simulink model "aar_generator"  (R2023a)
settings: Solver=FixedStepAuto  StartTime=0.0  StopTime=10  FixedStep=0.0001  RelTol=1e-3  AbsTol=1e-3
InitFcn:
  | addpath(fullfile(matlabroot,'toolbox/physmod/sm/sli/m'))
model workspace (MAT data in the model file):
  battery_cap = 1e-09
  contingency_time = 2
  final_demand = 1
  inertia_const = 0
  initial_amp = 0.91151
  max_torque = 1.1
  response_time = 0.05
  solar_cap = 1
  transmission_lim = 1000
undefined symbols (not defined in the file or in its folder): ee
libraries: fl_lib x141, ee_lib x60, nesl_utility x37, eeTransforms x12, batteryecm_lib x6, slpidlib x6, eeGeneralControl x6, eeSmAC1C x3, simulink x3, spsPLL3phLib x3
(part 3 of 4)

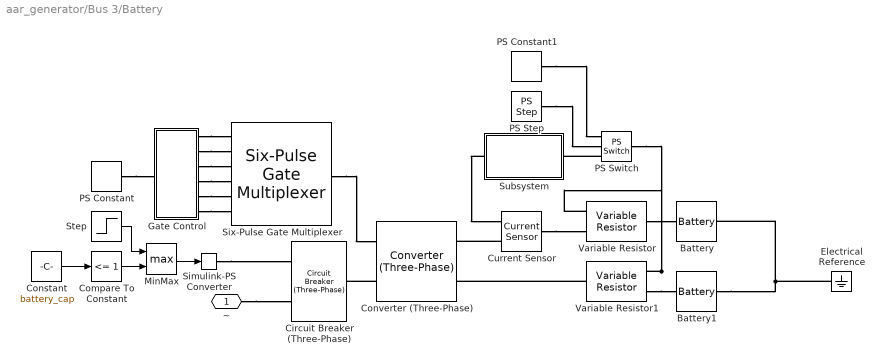
== system aar_generator/Bus 3/Battery ==
  Battery : batteryecm_lib/Battery  Vnom=494.97+50 kV  prm_dir=simscape.enum.battery.prm_dir.disabled  R1_dis=2 Ohm  R1_ch=2 Ohm  R1=0.17 Ohm  prm_AH=simscape.enum.battery.prm_AH.infinite  AH=50 A*hr  V1=11.5 V  AH1=25 A*hr  prm_R2=simscape.enum.battery.prm_R2.disabled  R2=2000 Ohm  Tmeas=298.15 K  charge_measurement_port=simscape.enum.battery.enable.no  prm_dyn=simscape.enum.battery.prm_dyn.off  Rp1=0.005 Ohm  tau1=30 s  Rp2=0.005 Ohm  tau2=30 s  Rp3=0.005 Ohm  tau3=30 s  Rp4=0.005 Ohm  tau4=30 s  Rp5=0.005 Ohm  tau5=30 s  prm_fade=simscape.enum.battery.prm_fade.disabled  N_fade=100  AH_fade=45 A*hr  R1_fade=2.02 Ohm  R1_ch_fade=2.02 Ohm  V1_fade=10.35 V  prm_age=simscape.enum.battery.prm_age.disabled  prm_age_OCV=simscape.enum.battery.prm_age_OCV.OCV  OCV_age=0.9  SOC_age=60  Tmeas_age=298.15 K  delta_time_age_vec=[0] d  temperature_age_vec=[273] K  OCV_scaling_age=2.2134e6  OCV_offset_age=1.632e6  temp_exp_age=0.515833569 V  t_exp_age=0.75  Vnom_T2=12 V  R1_T2=2.2 Ohm  R1_T2_dis=2.2 Ohm  R1_T2_ch=2.2 Ohm  V1_T2=11.4 V  R2_T2=2200 Ohm  Rp1_T2=0.005 Ohm  tau1_T2=30 s  Rp2_T2=0.005 Ohm  tau2_T2=30 s  Rp3_T2=0.005 Ohm  tau3_T2=30 s  Rp4_T2=0.005 Ohm  tau4_T2=30 s  Rp5_T2=0.005 Ohm  tau5_T2=30 s  Tmeas2=273.15 K  thermal_port=simscape.enum.thermaleffects.omit  thermal_mass=30000 J/K  i_specify=off  i_priority=None  i=0 A  i_nominal_specify=off  i_nominal_unit=A  i_nominal_value=1  v_specify=off  v_priority=None  v=0 V  v_nominal_specify=off  v_nominal_unit=V  v_nominal_value=1  charge_specify=off  charge_priority=High  charge=50 A*hr  charge_nominal_specify=off  charge_nominal_unit=A*hr  charge_nominal_value=1  num_cycles_specify=off  num_cycles_priority=High  num_cycles=0  num_cycles_nominal_specify=off  num_cycles_nominal_unit=1  num_cycles_nominal_value=1  temperature_specify=off  temperature_priority=High  temperature=298.15 K  temperature_nominal_specify=off  temperature_nominal_unit=K  temperature_nominal_value=1
  Battery1 : batteryecm_lib/Battery  Vnom=494.97+50 kV  prm_dir=simscape.enum.battery.prm_dir.disabled  R1_dis=2 Ohm  R1_ch=2 Ohm  R1=0.17 Ohm  prm_AH=simscape.enum.battery.prm_AH.infinite  AH=50 A*hr  V1=11.5 V  AH1=25 A*hr  prm_R2=simscape.enum.battery.prm_R2.disabled  R2=2000 Ohm  Tmeas=298.15 K  charge_measurement_port=simscape.enum.battery.enable.no  prm_dyn=simscape.enum.battery.prm_dyn.off  Rp1=0.005 Ohm  tau1=30 s  Rp2=0.005 Ohm  tau2=30 s  Rp3=0.005 Ohm  tau3=30 s  Rp4=0.005 Ohm  tau4=30 s  Rp5=0.005 Ohm  tau5=30 s  prm_fade=simscape.enum.battery.prm_fade.disabled  N_fade=100  AH_fade=45 A*hr  R1_fade=2.02 Ohm  R1_ch_fade=2.02 Ohm  V1_fade=10.35 V  prm_age=simscape.enum.battery.prm_age.disabled  prm_age_OCV=simscape.enum.battery.prm_age_OCV.OCV  OCV_age=0.9  SOC_age=60  Tmeas_age=298.15 K  delta_time_age_vec=[0] d  temperature_age_vec=[273] K  OCV_scaling_age=2.2134e6  OCV_offset_age=1.632e6  temp_exp_age=0.515833569 V  t_exp_age=0.75  Vnom_T2=12 V  R1_T2=2.2 Ohm  R1_T2_dis=2.2 Ohm  R1_T2_ch=2.2 Ohm  V1_T2=11.4 V  R2_T2=2200 Ohm  Rp1_T2=0.005 Ohm  tau1_T2=30 s  Rp2_T2=0.005 Ohm  tau2_T2=30 s  Rp3_T2=0.005 Ohm  tau3_T2=30 s  Rp4_T2=0.005 Ohm  tau4_T2=30 s  Rp5_T2=0.005 Ohm  tau5_T2=30 s  Tmeas2=273.15 K  thermal_port=simscape.enum.thermaleffects.omit  thermal_mass=30000 J/K  i_specify=off  i_priority=None  i=0 A  i_nominal_specify=off  i_nominal_unit=A  i_nominal_value=1  v_specify=off  v_priority=None  v=0 V  v_nominal_specify=off  v_nominal_unit=V  v_nominal_value=1  charge_specify=off  charge_priority=High  charge=50 A*hr  charge_nominal_specify=off  charge_nominal_unit=A*hr  charge_nominal_value=1  num_cycles_specify=off  num_cycles_priority=High  num_cycles=0  num_cycles_nominal_specify=off  num_cycles_nominal_unit=1  num_cycles_nominal_value=1  temperature_specify=off  temperature_priority=High  temperature=298.15 K  temperature_nominal_specify=off  temperature_nominal_unit=K  temperature_nominal_value=1
  Circuit Breaker (Three-Phase) : ee_lib/Switches & Breakers/Circuit Breaker (Three-Phase)  R_closed=1e-9 Ohm  G_open=1e-9 1/Ohm  threshold=0.5 V  breaker_behavior=ee.enum.switches.breakerBehavior.zeroCrossingEnable
      settings: InternalSimscapePortConfiguration="{\"Bottom\":[],\"Left\":[{\"id\":\"vT\",\"label\":\"vT\",\"type\":\"input\"},{\"id\":\"N1\",\"label\":\"~1\",\"type\":\"foundation.electrical.three_phase\"}],\"Right\":[{\"id\":\"N2\",\"label\":\"~2\",\"type\":\"foundation.electrical.three_phase\"}],\"Top\":[]}"
  Compare To Constant : simulink/Logic and Bit Operations/Compare To Constant  relop=<=  const=1  OutDataTypeStr=uint8
  Constant : Constant  Value=battery_cap
  Converter (Three-Phase) : ee_lib/Semiconductors & Converters/Converters/Converter (Three-Phase)  port_option=ee.enum.threePhasePort.composite  device_type=ee.enum.converters.switchingdevice.averaged  K=0  Vf=0.8 V  Ron=1e-9 mOhm  Rds=0.001 Ohm  Goff=1e-6 1/Ohm  Vgt=1 V  Vgt_off=-1 V  Ih=1 A  Vth=6 V  diode_param=ee.enum.converters.protectiondiode.none  diode_Vf=1 MV  diode_Ron=0.001 Ohm  diode_Goff=1e-5 1/Ohm  diode_C=50 nF  diode_iRM=-235 A  diode_iF=300 A  diode_idot=-50 A/us  diode_trr_param=ee.enum.converters.diodetrr.trr_factor  diode_trr_factor=3  diode_trr=15 us  diode_Qrr=1500 s*uA  snubber_type=ee.enum.converters.snubber.exclude  Cs=1e-7 F  Rs=0.1 Ohm
  Current Sensor : fl_lib/Electrical/Electrical Sensors/Current Sensor
  Electrical Reference : fl_lib/Electrical/Electrical Elements/Electrical Reference
  Gate Control : Subsystem
  MinMax : MinMax  Function=max  Inputs=2
  PS Constant : fl_lib/Physical Signals/Sources/PS Constant  constant=1
  PS Constant1 : fl_lib/Physical Signals/Sources/PS Constant  constant=0 Ohm
  PS Step : fl_lib/Physical Signals/Sources/PS Step  step_time=0.00025 s  initial_value=1  final_value=0
  PS Switch : fl_lib/Physical Signals/Nonlinear Operators/PS Switch  Threshold=0.5
      settings: InternalSimscapePortConfiguration="{\"Bottom\":[],\"Left\":[{\"id\":\"I1\",\"label\":\"\",\"type\":\"input\"},{\"id\":\"I2\",\"label\":\"\",\"type\":\"input\"},{\"id\":\"I3\",\"label\":\"\",\"type\":\"input\"}],\"Right\":[{\"id\":\"O\",\"label\":\"\",\"type\":\"output\"}],\"Top\":[]}"
  Simulink-PS Converter : nesl_utility/Simulink-PS Converter  PhysicalDomain=network_engine_domain  SubClassName=ps_input  LeftPortType=input  RightPortType=output  PseudoPeriodic=off  Frequencies=[]  NoiseDistribution=none  NoiseParameters=[]  Unit=V  AffineConversion=off  FilteringAndDerivatives=provide  SimscapeFilterOrder=1  InputFilterTimeConstant=0.001  UdotUserProvided=0
  Six-Pulse Gate Multiplexer : ee_lib/Semiconductors & Converters/Converters/Six-Pulse Gate Multiplexer  port_option=ee.enum.controlport.ps
  Step : Step  Time=contingency_time+response_time  Before=1  After=0  SampleTime=0
  Subsystem : Subsystem
  Variable Resistor : fl_lib/Electrical/Electrical Elements/Variable Resistor  Rmin=0 Ohm  i_specify=off  i_priority=None  i=0 A  i_nominal_specify=off  i_nominal_unit=A  i_nominal_value=1  v_specify=off  v_priority=None  v=0 V  v_nominal_specify=off  v_nominal_unit=V  v_nominal_value=1
  Variable Resistor1 : fl_lib/Electrical/Electrical Elements/Variable Resistor  Rmin=0 Ohm  i_specify=off  i_priority=None  i=0 A  i_nominal_specify=off  i_nominal_unit=A  i_nominal_value=1  v_specify=off  v_priority=None  v=0 V  v_nominal_specify=off  v_nominal_unit=V  v_nominal_value=1
  ~ : PMIOPort  Side=Left
  wires:
  Constant/1 -> Compare To Constant/1
  MinMax/1 -> Simulink-PS Converter/1
  Step/1 -> MinMax/1
  Compare To Constant/1 -> MinMax/2
  connections:
  PS Constant1/RConn1 -- PS Switch/LConn1
  PS Step/RConn1 -- PS Switch/LConn2
  Variable Resistor1/LConn1 -- Variable Resistor/LConn1 -- PS Switch/RConn1
  PS Switch/LConn3 -- Subsystem/RConn1
  Simulink-PS Converter/RConn1 -- Circuit Breaker (Three-Phase)/LConn1
  ~/RConn1 -- Circuit Breaker (Three-Phase)/LConn2
  Converter (Three-Phase)/LConn2 -- Circuit Breaker (Three-Phase)/RConn1
  Subsystem/LConn1 -- Current Sensor/RConn1
  Current Sensor/LConn1 -- Variable Resistor/LConn2
  Variable Resistor1/LConn2 -- Battery1/RConn1
  Variable Resistor1/RConn1 -- Converter (Three-Phase)/RConn2
  Variable Resistor/RConn1 -- Battery/LConn1
  Current Sensor/RConn2 -- Converter (Three-Phase)/RConn1
  Electrical Reference/LConn1 -- Battery/RConn1 -- Battery1/LConn1
  PS Constant/RConn1 -- Gate Control/LConn1
  Gate Control/RConn6 -- Six-Pulse Gate Multiplexer/LConn6
  Gate Control/RConn5 -- Six-Pulse Gate Multiplexer/LConn5
  Gate Control/RConn4 -- Six-Pulse Gate Multiplexer/LConn4
  Gate Control/RConn3 -- Six-Pulse Gate Multiplexer/LConn3
  Gate Control/RConn2 -- Six-Pulse Gate Multiplexer/LConn2
  Gate Control/RConn1 -- Six-Pulse Gate Multiplexer/LConn1
  Six-Pulse Gate Multiplexer/RConn1 -- Converter (Three-Phase)/LConn1

== system aar_generator/Bus 3/Governor and Prime Mover ==
  Governor : Subsystem
  Ideal Torque Source : fl_lib/Mechanical/Mechanical Sources/Ideal Torque Source
  Mechanical Rotational Reference : fl_lib/Mechanical/Rotational Elements/Mechanical Rotational Reference
  Non-reheat turbine : Subsystem
  PS-Simulink Converter : nesl_utility/PS-Simulink Converter  PhysicalDomain=network_engine_domain  SubClassName=ps_output  LeftPortType=input  RightPortType=output  PseudoPeriodic=off  Frequencies=[]  VectorFormat=1-D array  Unit=1  AffineConversion=off
  Rotor Velocity Measurement : ee_lib/Electromechanical/Synchronous/Synchronous Machine Measurement  output_idx=4
      settings: InternalSimscapePortConfiguration="{\"Bottom\":[],\"Left\":[{\"id\":\"pu_input\",\"label\":\"pu\",\"type\":\"input\"}],\"Right\":[{\"id\":\"pu_output\",\"label\":\"o\",\"type\":\"output\"}],\"Top\":[]}"
  Simulink-PS Converter : nesl_utility/Simulink-PS Converter  PhysicalDomain=network_engine_domain  SubClassName=ps_input  LeftPortType=input  RightPortType=output  PseudoPeriodic=off  Frequencies=[]  NoiseDistribution=none  NoiseParameters=[]  Unit=1  AffineConversion=off  FilteringAndDerivatives=zero  SimscapeFilterOrder=1  InputFilterTimeConstant=0.001  UdotUserProvided=1
  scale by base_torque : Gain  Gain=base_torque
  R : PMIOPort  Side=Right
  C : PMIOPort  Port=2  Side=Right
  pu : PMIOPort  Port=3  Side=Left
  wires:
  Non-reheat turbine/1(torque) -> scale by base_torque/1
  scale by base_torque/1 -> Simulink-PS Converter/1
  Governor/1(delta_y) -> Non-reheat turbine/1(delta_y)
  PS-Simulink Converter/1 -> Governor/1(pu_velocity)
  connections:
  Simulink-PS Converter/RConn1 -- Ideal Torque Source/RConn1
  PS-Simulink Converter/LConn1 -- Rotor Velocity Measurement/RConn1
  pu/RConn1 -- Rotor Velocity Measurement/LConn1
  Ideal Torque Source/LConn1 -- R/RConn1
  Mechanical Rotational Reference/LConn1 -- Ideal Torque Source/RConn2 -- C/RConn1

== system aar_generator/Bus 3/Load Control ==
  PS Gain : fl_lib/Physical Signals/Functions/PS Gain  gain=load MW
  PS Min : fl_lib/Physical Signals/Nonlinear Operators/PS Min
      settings: InternalSimscapePortConfiguration="{\"Bottom\":[],\"Left\":[{\"id\":\"I1\",\"label\":\"\",\"type\":\"input\"},{\"id\":\"I2\",\"label\":\"\",\"type\":\"input\"}],\"Right\":[{\"id\":\"O\",\"label\":\"\",\"type\":\"output\"}],\"Top\":[]}"
  PS Step : fl_lib/Physical Signals/Sources/PS Step  step_time=contingency_time+response_time s  initial_value=1  final_value=final_demand
  PS Step1 : fl_lib/Physical Signals/Sources/PS Step  step_time=0.15 s  initial_value=0.2  final_value=1
  Load (MW) : PMIOPort  Side=Right
  connections:
  PS Step1/RConn1 -- PS Min/LConn1
  PS Step/RConn1 -- PS Min/LConn2
  PS Min/RConn1 -- PS Gain/LConn1
  PS Gain/RConn1 -- Load (MW)/RConn1

== system aar_generator/Bus 3/Solar Panel ==
  Controlled Current Source (Three-Phase) : ee_lib/Sources/Controlled Current Source (Three-Phase)  input_option=ee.enum.inputType.instantaneous  FRated=60 Hz
      settings: InternalSimscapePortConfiguration="{\"Bottom\":[],\"Left\":[{\"id\":\"S\",\"label\":\"S\",\"type\":\"input\"},{\"id\":\"n\",\"label\":\"n\",\"type\":\"foundation.electrical.electrical\"}],\"Right\":[{\"id\":\"N\",\"label\":\"~\",\"type\":\"foundation.electrical.three_phase\"}],\"Top\":[]}"
  Current Control : Subsystem
  Electrical Reference : fl_lib/Electrical/Electrical Elements/Electrical Reference
  Grounded Neutral (Three-Phase) : ee_lib/Connectors & References/Grounded Neutral (Three-Phase)
  PS Step : fl_lib/Physical Signals/Sources/PS Step  step_time=0.15 s  initial_value=0  final_value=1
  Power Control : Subsystem
  Power Sensor (Three-Phase) : ee_lib/Sensors & Transducers/Power Sensor (Three-Phase)  load_type=ee.enum.passive.type_balanced.balanced  f0=60 Hz  config=ee.enum.with_neutral.no  rho=1
      settings: InternalSimscapePortConfiguration="{\"Bottom\":[],\"Left\":[{\"id\":\"N1\",\"label\":\"~1\",\"type\":\"foundation.electrical.three_phase\"}],\"Right\":[{\"id\":\"N2\",\"label\":\"~2\",\"type\":\"foundation.electrical.three_phase\"}],\"Top\":[{\"id\":\"Pm\",\"label\":\"P\",\"type\":\"output\"},{\"id\":\"Qm\",\"label\":\"Q\",\"type\":\"output\"}]}"
  SI to pu : Gain  Gain=1/(350*sqrt(2)*10^3)
  SPDT Switch (Three-Phase) : ee_lib/Switches & Breakers/SPDT Switch (Three-Phase)  R_closed=0.001 Ohm  G_open=1e-6 1/Ohm  threshold=0.5 V  i_vT_specify=off  i_vT_priority=None  i_vT=0 A  i_vT_nominal_specify=off  i_vT_nominal_unit=A  i_vT_nominal_value=1  I12_specify=off  I12_priority=None  I12=[0, 0, 0] A  I12_nominal_specify=off  I12_nominal_unit=A  I12_nominal_value=1  V12_specify=off  V12_priority=None  V12=[0, 0, 0] V  V12_nominal_specify=off  V12_nominal_unit=V  V12_nominal_value=1  I13_specify=off  I13_priority=None  I13=[0, 0, 0] A  I13_nominal_specify=off  I13_nominal_unit=A  I13_nominal_value=1  V13_specify=off  V13_priority=None  V13=[0, 0, 0] V  V13_nominal_specify=off  V13_nominal_unit=V  V13_nominal_value=1  i_a_12_specify=off  i_a_12_priority=None  i_a_12=0 A  i_a_12_nominal_specify=off  i_a_12_nominal_unit=A  i_a_12_nominal_value=1  v_a_12_specify=off  v_a_12_priority=None  v_a_12=0 V  v_a_12_nominal_specify=off  v_a_12_nominal_unit=V  v_a_12_nominal_value=1  i_a_13_specify=off  i_a_13_priority=None  i_a_13=0 A  i_a_13_nominal_specify=off  i_a_13_nominal_unit=A  i_a_13_nominal_value=1  v_a_13_specify=off  v_a_13_priority=None  v_a_13=0 V  v_a_13_nominal_specify=off  v_a_13_nominal_unit=V  v_a_13_nominal_value=1  i_b_12_specify=off  i_b_12_priority=None  i_b_12=0 A  i_b_12_nominal_specify=off  i_b_12_nominal_unit=A  i_b_12_nominal_value=1  v_b_12_specify=off  v_b_12_priority=None  v_b_12=0 V  v_b_12_nominal_specify=off  v_b_12_nominal_unit=V  v_b_12_nominal_value=1  i_b_13_specify=off  i_b_13_priority=None  i_b_13=0 A  i_b_13_nominal_specify=off  i_b_13_nominal_unit=A  i_b_13_nominal_value=1  v_b_13_specify=off  v_b_13_priority=None  v_b_13=0 V  v_b_13_nominal_specify=off  v_b_13_nominal_unit=V  v_b_13_nominal_value=1  i_c_12_specify=off  i_c_12_priority=None  i_c_12=0 A  i_c_12_nominal_specify=off  i_c_12_nominal_unit=A  i_c_12_nominal_value=1  v_c_12_specify=off  v_c_12_priority=None  v_c_12=0 V  v_c_12_nominal_specify=off  v_c_12_nominal_unit=V  v_c_12_nominal_value=1  i_c_13_specify=off  i_c_13_priority=None  i_c_13=0 A  i_c_13_nominal_specify=off  i_c_13_nominal_unit=A  i_c_13_nominal_value=1  v_c_13_specify=off  v_c_13_priority=None  v_c_13=0 V  v_c_13_nominal_specify=off  v_c_13_nominal_unit=V  v_c_13_nominal_value=1
      settings: InternalSimscapePortConfiguration="{\"Bottom\":[],\"Left\":[{\"id\":\"vT\",\"label\":\"vT\",\"type\":\"input\"},{\"id\":\"N1\",\"label\":\"~1\",\"type\":\"foundation.electrical.three_phase\"}],\"Right\":[{\"id\":\"N2\",\"label\":\"~2\",\"type\":\"foundation.electrical.three_phase\"},{\"id\":\"N3\",\"label\":\"~3\",\"type\":\"foundation.electrical.three_phase\"}],\"Top\":[]}"
  ~ : PMIOPort  Side=Left
  wires:
  [Phase3] -> Current Control/3(Phase)
  Power Control/2(Qset (pu)) -> Current Control/2(Qset (pu))
  [Freq3] -> Power Control/1(Freq (Hz))
  Power Control/1(Pset (pu)) -> Current Control/1(Pset (pu))
  [V3] -> SI to pu/1
  SI to pu/1 -> Current Control/4(Vabc (pu))
  connections:
  Current Control/RConn1 -- Controlled Current Source (Three-Phase)/LConn1
  Electrical Reference/LConn1 -- Controlled Current Source (Three-Phase)/LConn2
  Power Sensor (Three-Phase)/LConn1 -- Controlled Current Source (Three-Phase)/RConn1
  Power Control/LConn1 -- Power Sensor (Three-Phase)/LConn3
  ~/RConn1 -- SPDT Switch (Three-Phase)/RConn2
  PS Step/RConn1 -- SPDT Switch (Three-Phase)/LConn1
  SPDT Switch (Three-Phase)/LConn2 -- Power Sensor (Three-Phase)/RConn1
  Grounded Neutral (Three-Phase)/LConn1 -- SPDT Switch (Three-Phase)/RConn1

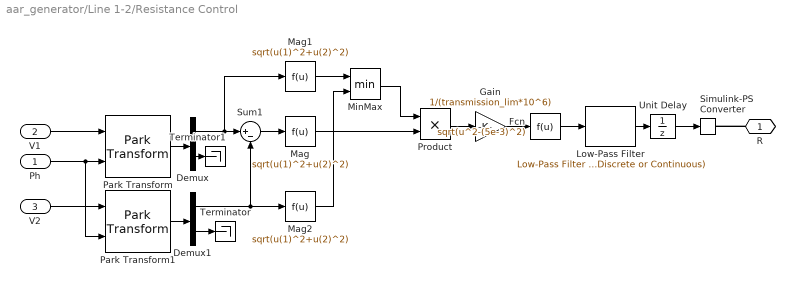
== system aar_generator/Line 1-2/Resistance Control ==
  Ph : Inport
  V1 : Inport  Port=2
  V2 : Inport  Port=3
  Demux : Demux  Outputs=[2 1]
  Demux1 : Demux  Outputs=[2 1]
  Fcn : Fcn  Expr=sqrt(u^2-(5e-3)^2)
  Gain : Gain  Gain=1/(transmission_lim*10^6)
  Low-Pass Filter : eeGeneralControl/Low-Pass Filter (Discrete or Continuous)  K=1  T=0.1  B=inf  A=-inf  init_option=Inherited from block input  x0=0  Ts=-1
  Mag : Fcn  Expr=sqrt(u(1)^2+u(2)^2)
  Mag1 : Fcn  Expr=sqrt(u(1)^2+u(2)^2)
  Mag2 : Fcn  Expr=sqrt(u(1)^2+u(2)^2)
  MinMax : MinMax  Inputs=2
  Park Transform : eeTransforms/Park Transform  AxisAlignment=Q-axis  PowerInvariant=off
      settings: LibrarySourceBlock=|
      | ee_sl_lib/Mathematical
      | Transforms/Park Transform
  Park Transform1 : eeTransforms/Park Transform  AxisAlignment=Q-axis  PowerInvariant=off
      settings: LibrarySourceBlock=|
      | ee_sl_lib/Mathematical
      | Transforms/Park Transform
  Product : Product
  Simulink-PS Converter : nesl_utility/Simulink-PS Converter  PhysicalDomain=network_engine_domain  SubClassName=ps_input  LeftPortType=input  RightPortType=output  PseudoPeriodic=off  Frequencies=[]  NoiseDistribution=none  NoiseParameters=[]  Unit=Ohm  AffineConversion=off  FilteringAndDerivatives=provide  SimscapeFilterOrder=1  InputFilterTimeConstant=0.001  UdotUserProvided=0
  Sum1 : Sum  Inputs=|+-
  Terminator : Terminator
  Terminator1 : Terminator
  Unit Delay : UnitDelay  SampleTime=-1  HasFrameUpgradeWarning=on
  R : PMIOPort  Side=Right
  wires:
  Unit Delay/1 -> Simulink-PS Converter/1
  V1/1 -> Park Transform/1
  V2/1 -> Park Transform1/1
  Ph/1 -> Park Transform1/2, Park Transform/2
  Park Transform/1 -> Demux/1
  Park Transform1/1 -> Demux1/1
  Demux1/2 -> Terminator/1
  Demux/2 -> Terminator1/1
  Demux/1 -> Mag1/1, Sum1/1
  Demux1/1 -> Mag2/1, Sum1/2
  Sum1/1 -> Mag/1
  Mag1/1 -> MinMax/1
  Mag2/1 -> MinMax/2
  Mag/1 -> Product/2
  MinMax/1 -> Product/1
  Product/1 -> Gain/1
  Low-Pass Filter/1 -> Unit Delay/1
  Gain/1 -> Fcn/1
  Fcn/1 -> Low-Pass Filter/1
  connections:
  R/RConn1 -- Simulink-PS Converter/RConn1

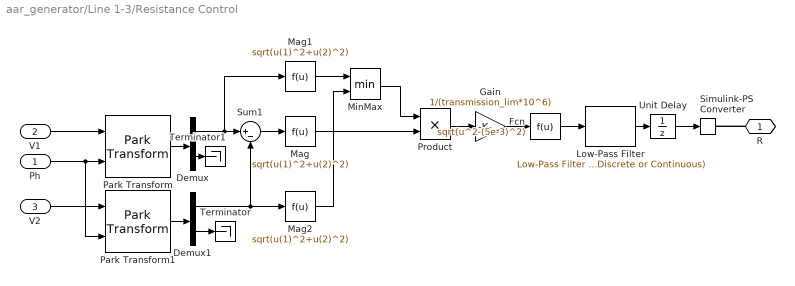
== system aar_generator/Line 1-3/Resistance Control ==
  Ph : Inport
  V1 : Inport  Port=2
  V2 : Inport  Port=3
  Demux : Demux  Outputs=[2 1]
  Demux1 : Demux  Outputs=[2 1]
  Fcn : Fcn  Expr=sqrt(u^2-(5e-3)^2)
  Gain : Gain  Gain=1/(transmission_lim*10^6)
  Low-Pass Filter : eeGeneralControl/Low-Pass Filter (Discrete or Continuous)  K=1  T=0.1  B=inf  A=-inf  init_option=Inherited from block input  x0=0  Ts=-1
  Mag : Fcn  Expr=sqrt(u(1)^2+u(2)^2)
  Mag1 : Fcn  Expr=sqrt(u(1)^2+u(2)^2)
  Mag2 : Fcn  Expr=sqrt(u(1)^2+u(2)^2)
  MinMax : MinMax  Inputs=2
  Park Transform : eeTransforms/Park Transform  AxisAlignment=Q-axis  PowerInvariant=off
      settings: LibrarySourceBlock=|
      | ee_sl_lib/Mathematical
      | Transforms/Park Transform
  Park Transform1 : eeTransforms/Park Transform  AxisAlignment=Q-axis  PowerInvariant=off
      settings: LibrarySourceBlock=|
      | ee_sl_lib/Mathematical
      | Transforms/Park Transform
  Product : Product
  Simulink-PS Converter : nesl_utility/Simulink-PS Converter  PhysicalDomain=network_engine_domain  SubClassName=ps_input  LeftPortType=input  RightPortType=output  PseudoPeriodic=off  Frequencies=[]  NoiseDistribution=none  NoiseParameters=[]  Unit=Ohm  AffineConversion=off  FilteringAndDerivatives=provide  SimscapeFilterOrder=1  InputFilterTimeConstant=0.001  UdotUserProvided=0
  Sum1 : Sum  Inputs=|+-
  Terminator : Terminator
  Terminator1 : Terminator
  Unit Delay : UnitDelay  SampleTime=-1  HasFrameUpgradeWarning=on
  R : PMIOPort  Side=Right
  wires:
  Unit Delay/1 -> Simulink-PS Converter/1
  V1/1 -> Park Transform/1
  V2/1 -> Park Transform1/1
  Ph/1 -> Park Transform1/2, Park Transform/2
  Park Transform/1 -> Demux/1
  Park Transform1/1 -> Demux1/1
  Demux1/2 -> Terminator/1
  Demux/2 -> Terminator1/1
  Demux/1 -> Mag1/1, Sum1/1
  Demux1/1 -> Mag2/1, Sum1/2
  Sum1/1 -> Mag/1
  Mag1/1 -> MinMax/1
  Mag2/1 -> MinMax/2
  Mag/1 -> Product/2
  MinMax/1 -> Product/1
  Product/1 -> Gain/1
  Low-Pass Filter/1 -> Unit Delay/1
  Gain/1 -> Fcn/1
  Fcn/1 -> Low-Pass Filter/1
  connections:
  R/RConn1 -- Simulink-PS Converter/RConn1

== system aar_generator/Line 2-3/Resistance Control ==
  Ph : Inport
  V1 : Inport  Port=2
  V2 : Inport  Port=3
  Demux : Demux  Outputs=[2 1]
  Demux1 : Demux  Outputs=[2 1]
  Fcn : Fcn  Expr=sqrt(u^2-(5e-3)^2)
  Gain : Gain  Gain=1/(transmission_lim*10^6)
  Low-Pass Filter : eeGeneralControl/Low-Pass Filter (Discrete or Continuous)  K=1  T=0.1  B=inf  A=-inf  init_option=Inherited from block input  x0=0  Ts=-1
  Mag : Fcn  Expr=sqrt(u(1)^2+u(2)^2)
  Mag1 : Fcn  Expr=sqrt(u(1)^2+u(2)^2)
  Mag2 : Fcn  Expr=sqrt(u(1)^2+u(2)^2)
  MinMax : MinMax  Inputs=2
  Park Transform : eeTransforms/Park Transform  AxisAlignment=Q-axis  PowerInvariant=off
      settings: LibrarySourceBlock=|
      | ee_sl_lib/Mathematical
      | Transforms/Park Transform
  Park Transform1 : eeTransforms/Park Transform  AxisAlignment=Q-axis  PowerInvariant=off
      settings: LibrarySourceBlock=|
      | ee_sl_lib/Mathematical
      | Transforms/Park Transform
  Product : Product
  Simulink-PS Converter : nesl_utility/Simulink-PS Converter  PhysicalDomain=network_engine_domain  SubClassName=ps_input  LeftPortType=input  RightPortType=output  PseudoPeriodic=off  Frequencies=[]  NoiseDistribution=none  NoiseParameters=[]  Unit=Ohm  AffineConversion=off  FilteringAndDerivatives=provide  SimscapeFilterOrder=1  InputFilterTimeConstant=0.001  UdotUserProvided=0
  Sum1 : Sum  Inputs=|+-
  Terminator : Terminator
  Terminator1 : Terminator
  Unit Delay : UnitDelay  SampleTime=-1  HasFrameUpgradeWarning=on
  R : PMIOPort  Side=Right
  wires:
  Unit Delay/1 -> Simulink-PS Converter/1
  V1/1 -> Park Transform/1
  V2/1 -> Park Transform1/1
  Ph/1 -> Park Transform1/2, Park Transform/2
  Park Transform/1 -> Demux/1
  Park Transform1/1 -> Demux1/1
  Demux1/2 -> Terminator/1
  Demux/2 -> Terminator1/1
  Demux/1 -> Mag1/1, Sum1/1
  Demux1/1 -> Mag2/1, Sum1/2
  Sum1/1 -> Mag/1
  Mag1/1 -> MinMax/1
  Mag2/1 -> MinMax/2
  Mag/1 -> Product/2
  MinMax/1 -> Product/1
  Product/1 -> Gain/1
  Low-Pass Filter/1 -> Unit Delay/1
  Gain/1 -> Fcn/1
  Fcn/1 -> Low-Pass Filter/1
  connections:
  R/RConn1 -- Simulink-PS Converter/RConn1

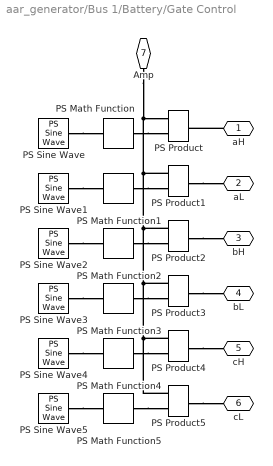
== system aar_generator/Bus 1/Battery/Gate Control ==
  PS Math Function{,1..5} (6 alike) : fl_lib/Physical Signals/Functions/PS Math Function  fcn_choice=foundation.enum.math_function.square  v=1
  PS Product{,1..5} (6 alike) : fl_lib/Physical Signals/Functions/PS Product
  PS Sine Wave : fl_lib/Physical Signals/Sources/PS Sine Wave  amplitude=1  bias=0  frequency_spec=foundation.enum.frequencySpec.frequencySI  frequency_SI=30 Hz  frequency_angular=1 rad/s  phase=pi/2 rad
      settings: InternalSimscapePortConfiguration="{\"Bottom\":[],\"Left\":[],\"Right\":[{\"id\":\"O\",\"label\":\"\",\"type\":\"output\"}],\"Top\":[]}"
  PS Sine Wave1 : fl_lib/Physical Signals/Sources/PS Sine Wave  amplitude=1  bias=0  frequency_spec=foundation.enum.frequencySpec.frequencySI  frequency_SI=30 Hz  frequency_angular=1 rad/s  phase=0 rad
      settings: InternalSimscapePortConfiguration="{\"Bottom\":[],\"Left\":[],\"Right\":[{\"id\":\"O\",\"label\":\"\",\"type\":\"output\"}],\"Top\":[]}"
  PS Sine Wave2 : fl_lib/Physical Signals/Sources/PS Sine Wave  amplitude=1  bias=0  frequency_spec=foundation.enum.frequencySpec.frequencySI  frequency_SI=30 Hz  frequency_angular=1 rad/s  phase=2*pi/3+pi/2 rad
      settings: InternalSimscapePortConfiguration="{\"Bottom\":[],\"Left\":[],\"Right\":[{\"id\":\"O\",\"label\":\"\",\"type\":\"output\"}],\"Top\":[]}"
  PS Sine Wave3 : fl_lib/Physical Signals/Sources/PS Sine Wave  amplitude=1  bias=0  frequency_spec=foundation.enum.frequencySpec.frequencySI  frequency_SI=30 Hz  frequency_angular=1 rad/s  phase=2*pi/3 rad
      settings: InternalSimscapePortConfiguration="{\"Bottom\":[],\"Left\":[],\"Right\":[{\"id\":\"O\",\"label\":\"\",\"type\":\"output\"}],\"Top\":[]}"
  PS Sine Wave4 : fl_lib/Physical Signals/Sources/PS Sine Wave  amplitude=1  bias=0  frequency_spec=foundation.enum.frequencySpec.frequencySI  frequency_SI=30 Hz  frequency_angular=1 rad/s  phase=-2*pi/3+pi/2 rad
      settings: InternalSimscapePortConfiguration="{\"Bottom\":[],\"Left\":[],\"Right\":[{\"id\":\"O\",\"label\":\"\",\"type\":\"output\"}],\"Top\":[]}"
  PS Sine Wave5 : fl_lib/Physical Signals/Sources/PS Sine Wave  amplitude=1  bias=0  frequency_spec=foundation.enum.frequencySpec.frequencySI  frequency_SI=30 Hz  frequency_angular=1 rad/s  phase=-2*pi/3 rad
      settings: InternalSimscapePortConfiguration="{\"Bottom\":[],\"Left\":[],\"Right\":[{\"id\":\"O\",\"label\":\"\",\"type\":\"output\"}],\"Top\":[]}"
  aH : PMIOPort  Side=Right
  aL : PMIOPort  Port=2  Side=Right
  bH : PMIOPort  Port=3  Side=Right
  bL : PMIOPort  Port=4  Side=Right
  cH : PMIOPort  Port=5  Side=Right
  cL : PMIOPort  Port=6  Side=Right
  Amp : PMIOPort  Port=7  Side=Left
  connections:
  aH/RConn1 -- PS Product/RConn1
  PS Math Function/RConn1 -- PS Product/LConn2
  Amp/RConn1 -- PS Product/LConn1 -- PS Product1/LConn1 -- PS Product2/LConn1 -- PS Product3/LConn1 -- PS Product5/LConn1 -- PS Product4/LConn1
  PS Sine Wave/RConn1 -- PS Math Function/LConn1
  PS Math Function1/RConn1 -- PS Product1/LConn2
  PS Sine Wave1/RConn1 -- PS Math Function1/LConn1
  PS Product1/RConn1 -- aL/RConn1
  PS Math Function2/RConn1 -- PS Product2/LConn2
  PS Sine Wave2/RConn1 -- PS Math Function2/LConn1
  PS Product2/RConn1 -- bH/RConn1
  PS Math Function3/RConn1 -- PS Product3/LConn2
  PS Sine Wave3/RConn1 -- PS Math Function3/LConn1
  PS Product3/RConn1 -- bL/RConn1
  PS Math Function4/RConn1 -- PS Product4/LConn2
  PS Sine Wave4/RConn1 -- PS Math Function4/LConn1
  PS Math Function5/RConn1 -- PS Product5/LConn2
  PS Sine Wave5/RConn1 -- PS Math Function5/LConn1
  PS Product4/RConn1 -- cH/RConn1
  PS Product5/RConn1 -- cL/RConn1

== system aar_generator/Bus 1/Battery/Subsystem ==
  Internal Resistance : fl_lib/Physical Signals/Sources/PS Constant  constant=0.34 Ohm
  PS Add : fl_lib/Physical Signals/Functions/PS Add
  PS Gain1 : fl_lib/Physical Signals/Functions/PS Gain  gain=0.5
  PS Gain2 : fl_lib/Physical Signals/Functions/PS Gain  gain=battery_cap MW
  PS Gain3 : fl_lib/Physical Signals/Functions/PS Gain  gain=2*350*sqrt(2) kV
  PS Math Function : fl_lib/Physical Signals/Functions/PS Math Function  fcn_choice=foundation.enum.math_function.square  v=1
  PS Math Function1 : fl_lib/Physical Signals/Functions/PS Math Function  fcn_choice=foundation.enum.math_function.reciprocal  v=1
  PS Subtract : fl_lib/Physical Signals/Functions/PS Subtract
  I : PMIOPort  Side=Left
  r : PMIOPort  Port=2  Side=Right
  connections:
  I/RConn1 -- PS Math Function1/LConn1
  PS Gain1/LConn1 -- PS Subtract/RConn1
  PS Gain1/RConn1 -- r/RConn1
  PS Add/RConn1 -- PS Subtract/LConn2
  Internal Resistance/RConn1 -- PS Add/LConn2
  PS Math Function1/RConn1 -- PS Math Function/LConn1 -- PS Gain3/LConn1
  PS Gain2/LConn1 -- PS Math Function/RConn1
  PS Add/LConn1 -- PS Gain2/RConn1
  PS Gain3/RConn1 -- PS Subtract/LConn1

== system aar_generator/Bus 1/Governor and Prime Mover/Governor ==
  pu_velocity : Inport
  1/T_G : Gain  Gain=1/T_G
  1/droop : Gain  Gain=1/(droop_percentage/100)
  Delta load setpoint : Sum  Inputs=+-|
  Delta speed : Sum  Inputs=-+|
  Integrator : Integrator  InitialCondition=pu_torque0
  Load_setpoint : Constant  Value=pu_load_reference_setpoint
  Speed_ref : Constant  Value=pu_speed_reference
  Subtract : Sum  Inputs=|+-
  delta_y : Outport  VectorParamsAs1DForOutWhenUnconnected=off
  wires:
  Speed_ref/1 -> Delta speed/1
  Delta speed/1 -> 1/droop/1
  Load_setpoint/1 -> Delta load setpoint/1
  pu_velocity/1 -> Delta speed/2
  1/droop/1 -> Delta load setpoint/2
  Delta load setpoint/1 -> Subtract/1
  Subtract/1 -> 1/T_G/1
  1/T_G/1 -> Integrator/1
  Integrator/1 -> delta_y/1, Subtract/2

== system aar_generator/Bus 1/Governor and Prime Mover/Non-reheat turbine ==
  delta_y : Inport
  1/T_CH : Gain  Gain=1/T_CH
  Integrator : Integrator  InitialCondition=pu_torque0  UpperSaturationLimit=max_torque
  Max : MinMax  Function=max  Inputs=2
  Min : MinMax  Inputs=2
  Step : Step  Time=contingency_time  Before=max_torque  After=contingency_torque  SampleTime=0
  Sum : Sum  Inputs=|+-
  has_contingency : Constant  Value=max_torque*(1-has_contingency)
  torque : Outport  VectorParamsAs1DForOutWhenUnconnected=off
  wires:
  delta_y/1 -> Sum/1
  Sum/1 -> 1/T_CH/1
  1/T_CH/1 -> Integrator/1
  Min/1 -> Sum/2, torque/1
  Integrator/1 -> Min/2
  Max/1 -> Min/1
  Step/1 -> Max/2
  has_contingency/1 -> Max/1

== system aar_generator/Bus 1/Solar Panel/Current Control ==
  Pset (pu) : Inport
  Qset (pu) : Inport  Port=2
  Phase : Inport  Port=3
  Vabc (pu) : Inport  Port=4
  Constant : Constant  Value=0
  Demux : Demux  Outputs=[2 1]
  Divide : Product  Inputs=*/
  Id : Fcn  Expr=u(1)*u(3)+u(2)*u(4)
  Inverse Park Transform : eeTransforms/Inverse Park Transform  AxisAlignment=Q-axis  PowerInvariant=off
      settings: LibrarySourceBlock=|
      | ee_sl_lib/Mathematical
      | Transforms/Inverse
      | Park Transform
  Iq : Fcn  Expr=u(1)*u(4)-u(2)*u(3)
  Mag^2 : Fcn  Expr=u(1)^2+u(2)^2
  Mux : Mux  Inputs=3
  Mux1 : Mux  Inputs=3
  Park Transform : eeTransforms/Park Transform  AxisAlignment=Q-axis  PowerInvariant=off
      settings: LibrarySourceBlock=|
      | ee_sl_lib/Mathematical
      | Transforms/Park Transform
  Simulink-PS Converter : nesl_utility/Simulink-PS Converter  PhysicalDomain=network_engine_domain  SubClassName=ps_input  LeftPortType=input  RightPortType=output  PseudoPeriodic=off  Frequencies=[]  NoiseDistribution=none  NoiseParameters=[]  Unit=A  AffineConversion=off  FilteringAndDerivatives=filter  SimscapeFilterOrder=1  InputFilterTimeConstant=0.0001  UdotUserProvided=0
  Terminator : Terminator
  Unit Delay1 : UnitDelay  InitialCondition=[0 -sin(2*pi/3) sin(2*pi/3)]  SampleTime=-1  HasFrameUpgradeWarning=on
  pu to SI : Gain  Gain=1/3*0.8*load/350*10^3*sqrt(2)
  Iabc (SI) : PMIOPort  Side=Right
  wires:
  Park Transform/1 -> Demux/1
  Demux/2 -> Terminator/1
  Demux/1 -> Mux/3, Mag^2/1
  Mag^2/1 -> Divide/2
  pu to SI/1 -> Simulink-PS Converter/1
  Constant/1 -> Mux1/3
  Phase/1 -> Inverse Park Transform/2, Park Transform/2
  Vabc (pu)/1 -> Park Transform/1
  Id/1 -> Mux1/1
  Iq/1 -> Mux1/2
  Inverse Park Transform/1 -> Unit Delay1/1
  Unit Delay1/1 -> pu to SI/1
  Mux1/1 -> Divide/1
  Divide/1 -> Inverse Park Transform/1
  Pset (pu)/1 -> Mux/1
  Qset (pu)/1 -> Mux/2
  Mux/1 -> Id/1, Iq/1
  connections:
  Iabc (SI)/RConn1 -- Simulink-PS Converter/RConn1

== system aar_generator/Bus 1/Solar Panel/Power Control ==
  Freq (Hz) : Inport
  Discrete PID Controller : slpidlib/PID Controller  Controller=PID  Form=Parallel  TimeDomain=Discrete-time  UseExternalTs=off  SampleTime=-1  IntegratorMethod=Forward Euler  FilterMethod=Forward Euler  ControllerParametersSource=internal  P=5  I=100  UseKiTs=off  D=0  N=100  UseFilter=on  TunerSelectOption=Transfer Function Based (PID Tuner App)  InitialConditionSource=internal  InitialConditionForIntegrator=0  InitialConditionForFilter=0  DifferentiatorICPrevScaledInput=0  ExternalReset=none  TrackingMode=off  Kt=1  LimitOutput=off  SatLimitsSource=internal  UpperSaturationLimit=inf  LowerSaturationLimit=-inf  LinearizeAsGain=off  AntiWindupMode=none  Kb=1  LimitIntegrator=off  UpperIntegratorSaturationLimit=inf  LowerIntegratorSaturationLimit=-inf  POutMin=[]  POutMax=[]  IOutMin=[]  IOutMax=[]  DOutMin=[]  DOutMax=[]  NOutMin=[]  NOutMax=[]  SumOutMin=[]  SumOutMax=[]  SaturationOutMin=[]  SaturationOutMax=[]  PParamMin=[]  PParamMax=[]  IParamMin=[]  IParamMax=[]  DParamMin=[]  DParamMax=[]  NParamMin=[]  NParamMax=[]  KbParamMin=[]  KbParamMax=[]  KtParamMin=[]  KtParamMax=[]  KbOutMin=[]  KbOutMax=[]  KtOutMin=[]  KtOutMax=[]  IntegratorOutMin=[]  IntegratorOutMax=[]  FilterOutMin=[]  FilterOutMax=[]  SumI1OutMin=[]  SumI1OutMax=[]  SumI2OutMin=[]  SumI2OutMax=[]  SumI3OutMin=[]  SumI3OutMax=[]  SumI4OutMin=[]  SumI4OutMax=[]  SumDOutMin=[]  SumDOutMax=[]  DifferentiatorOutMin=[]  DifferentiatorOutMax=[]  FilterDiffOutCoefMin=[]  FilterDiffOutCoefMax=[]  ReciprocalOutMin=[]  ReciprocalOutMax=[]  SumDenOutMin=[]  SumDenOutMax=[]  SumNumOutMin=[]  SumNumOutMax=[]  DivideOutMin=[]  DivideOutMax=[]  UdiffTsProdOutMin=[]  UdiffTsProdOutMax=[]  NTsProdOutMin=[]  NTsProdOutMax=[]  UintegralTsProdOutMin=[]  UintegralTsProdOutMax=[]  UngainTsProdOutMin=[]  UngainTsProdOutMax=[]  ClampingZeroOutDataTypeStr=Inherit: Inherit via back propagation  ClampingZeroOutMin=[]  ClampingZeroOutMax=[]  FilterDenConstantOutDataTypeStr=Inherit: Inherit via back propagation  FilterDenConstantOutMin=[]  FilterDenConstantOutMax=[]  PCopyOutDataTypeStr=Inherit: Inherit via back propagation  PCopyOutMin=[]  PCopyOutMax=[]  NCopyOutDataTypeStr=Inherit: Inherit via back propagation  NCopyOutMin=[]  NCopyOutMax=[]  IntegratorContinuousStateAttributes=''  IntegratorStateMustResolveToSignalObject=off  IntegratorRTWStateStorageClass=Auto  FilterContinuousStateAttributes=''  FilterStateMustResolveToSignalObject=off  FilterRTWStateStorageClass=Auto  ParallelPVariant=InternalParameters  IdealPVariant=Disabled  IVariant=InternalParameters  DVariant=InternalParameters  IntegratorVariant=Discrete  SatVariant=Disabled  AWVariant=Passthrough  PCopyVariant=Disabled  TRVariant=Disabled  FdbkBlocksVariant=Forward  IdealPFdbkVariant=Disabled  SatFdbkVariant=Disabled  DerivativeFilterVariant=ForwardEulerFilter  NVariant=InternalParameters  NCopyVariant=Disabled  FilterICVariant=InternalICsFilter  IntegratorICVariant=InternalICs  ExternalResetVariant=Disabled  TRSumVariant=Passthrough  SumFdbkVariant=Disabled  SumVariant=Sum_PID  TsampFilterVariant=InternalTs  TsampNgainVariant=Passthrough  TsampIntegralVariant=Disabled_SignalSpec  ExternalSaturationOutDataTypeStr=Inherit: Same as second input
      settings: LibrarySourceBlock=simulink/Discrete/Discrete PID Controller
  Discrete PID Controller1 : slpidlib/PID Controller  Controller=PID  Form=Parallel  TimeDomain=Discrete-time  UseExternalTs=off  SampleTime=-1  IntegratorMethod=Forward Euler  FilterMethod=Forward Euler  ControllerParametersSource=internal  P=20  I=20  UseKiTs=off  D=0  N=100  UseFilter=on  TunerSelectOption=Transfer Function Based (PID Tuner App)  InitialConditionSource=internal  InitialConditionForIntegrator=0  InitialConditionForFilter=0  DifferentiatorICPrevScaledInput=0  ExternalReset=none  TrackingMode=off  Kt=1  LimitOutput=on  SatLimitsSource=internal  UpperSaturationLimit=1  LowerSaturationLimit=1-solar_cap  LinearizeAsGain=off  AntiWindupMode=clamping  Kb=1  LimitIntegrator=off  UpperIntegratorSaturationLimit=inf  LowerIntegratorSaturationLimit=-inf  POutMin=[]  POutMax=[]  IOutMin=[]  IOutMax=[]  DOutMin=[]  DOutMax=[]  NOutMin=[]  NOutMax=[]  SumOutMin=[]  SumOutMax=[]  SaturationOutMin=[]  SaturationOutMax=[]  PParamMin=[]  PParamMax=[]  IParamMin=[]  IParamMax=[]  DParamMin=[]  DParamMax=[]  NParamMin=[]  NParamMax=[]  KbParamMin=[]  KbParamMax=[]  KtParamMin=[]  KtParamMax=[]  KbOutMin=[]  KbOutMax=[]  KtOutMin=[]  KtOutMax=[]  IntegratorOutMin=[]  IntegratorOutMax=[]  FilterOutMin=[]  FilterOutMax=[]  SumI1OutMin=[]  SumI1OutMax=[]  SumI2OutMin=[]  SumI2OutMax=[]  SumI3OutMin=[]  SumI3OutMax=[]  SumI4OutMin=[]  SumI4OutMax=[]  SumDOutMin=[]  SumDOutMax=[]  DifferentiatorOutMin=[]  DifferentiatorOutMax=[]  FilterDiffOutCoefMin=[]  FilterDiffOutCoefMax=[]  ReciprocalOutMin=[]  ReciprocalOutMax=[]  SumDenOutMin=[]  SumDenOutMax=[]  SumNumOutMin=[]  SumNumOutMax=[]  DivideOutMin=[]  DivideOutMax=[]  UdiffTsProdOutMin=[]  UdiffTsProdOutMax=[]  NTsProdOutMin=[]  NTsProdOutMax=[]  UintegralTsProdOutMin=[]  UintegralTsProdOutMax=[]  UngainTsProdOutMin=[]  UngainTsProdOutMax=[]  ClampingZeroOutDataTypeStr=Inherit: Inherit via back propagation  ClampingZeroOutMin=[]  ClampingZeroOutMax=[]  FilterDenConstantOutDataTypeStr=Inherit: Inherit via back propagation  FilterDenConstantOutMin=[]  FilterDenConstantOutMax=[]  PCopyOutDataTypeStr=Inherit: Inherit via back propagation  PCopyOutMin=[]  PCopyOutMax=[]  NCopyOutDataTypeStr=Inherit: Inherit via back propagation  NCopyOutMin=[]  NCopyOutMax=[]  IntegratorContinuousStateAttributes=''  IntegratorStateMustResolveToSignalObject=off  IntegratorRTWStateStorageClass=Auto  FilterContinuousStateAttributes=''  FilterStateMustResolveToSignalObject=off  FilterRTWStateStorageClass=Auto  ParallelPVariant=InternalParameters  IdealPVariant=Disabled  IVariant=InternalParameters  DVariant=InternalParameters  IntegratorVariant=Discrete  SatVariant=Enabled  AWVariant=DiscClampingParallel  PCopyVariant=Disabled  TRVariant=Disabled  FdbkBlocksVariant=Forward  IdealPFdbkVariant=Disabled  SatFdbkVariant=Disabled  DerivativeFilterVariant=ForwardEulerFilter  NVariant=InternalParameters  NCopyVariant=Disabled  FilterICVariant=InternalICsFilter  IntegratorICVariant=InternalICs  ExternalResetVariant=Disabled  TRSumVariant=Passthrough  SumFdbkVariant=Disabled  SumVariant=Sum_PID  TsampFilterVariant=InternalTs  TsampNgainVariant=Passthrough  TsampIntegralVariant=Disabled_SignalSpec  ExternalSaturationOutDataTypeStr=Inherit: Same as second input
      settings: LibrarySourceBlock=simulink/Discrete/Discrete PID Controller
  Gain : Gain  Gain=-1
  Load Set : Constant
  Low-Pass Filter (Discrete or Continuous) : eeGeneralControl/Low-Pass Filter (Discrete or Continuous)  K=1  T=0.1  B=inf  A=-inf  init_option=Inherited from block input  x0=0  Ts=-1
  PS-Simulink Converter : nesl_utility/PS-Simulink Converter  PhysicalDomain=network_engine_domain  SubClassName=ps_output  LeftPortType=input  RightPortType=output  PseudoPeriodic=off  Frequencies=[]  VectorFormat=inherit  Unit=inherit  AffineConversion=off
  Rate Limiter : RateLimiter  RisingSlewLimit=5  FallingSlewLimit=-5  SampleTimeMode=inherited  InitialCondition=1
  Ref Freq : Constant
  SI to pu : Gain  Gain=1/60
  SI to pu1 : Gain  Gain=1/(0.8*load*10^6)
  Sum : Sum  Inputs=-+|
  Sum1 : Sum  Inputs=+-|
  Q (SI) : PMIOPort  Side=Left
  Pset (pu) : Outport
  Qset (pu) : Outport  Port=2
  wires:
  SI to pu1/1 -> Gain/1
  Gain/1 -> Discrete PID Controller/1
  PS-Simulink Converter/1 -> SI to pu1/1
  Freq (Hz)/1 -> SI to pu/1
  SI to pu/1 -> Sum/2
  Ref Freq/1 -> Sum/1
  Load Set/1 -> Sum1/1
  Sum/1 -> Discrete PID Controller1/1
  Discrete PID Controller1/1 -> Sum1/2
  Sum1/1 -> Rate Limiter/1
  Rate Limiter/1 -> Pset (pu)/1
  Discrete PID Controller/1 -> Low-Pass Filter (Discrete or Continuous)/1
  Low-Pass Filter (Discrete or Continuous)/1 -> Qset (pu)/1
  connections:
  Q (SI)/RConn1 -- PS-Simulink Converter/LConn1

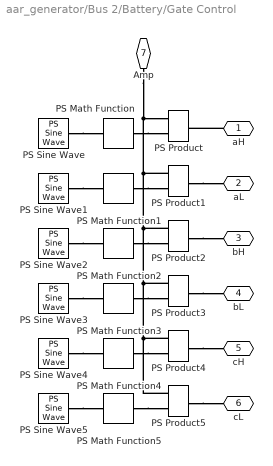
== system aar_generator/Bus 2/Battery/Gate Control ==
  PS Math Function{,1..5} (6 alike) : fl_lib/Physical Signals/Functions/PS Math Function  fcn_choice=foundation.enum.math_function.square  v=1
  PS Product{,1..5} (6 alike) : fl_lib/Physical Signals/Functions/PS Product
  PS Sine Wave : fl_lib/Physical Signals/Sources/PS Sine Wave  amplitude=1  bias=0  frequency_spec=foundation.enum.frequencySpec.frequencySI  frequency_SI=30 Hz  frequency_angular=1 rad/s  phase=pi/2 rad
      settings: InternalSimscapePortConfiguration="{\"Bottom\":[],\"Left\":[],\"Right\":[{\"id\":\"O\",\"label\":\"\",\"type\":\"output\"}],\"Top\":[]}"
  PS Sine Wave1 : fl_lib/Physical Signals/Sources/PS Sine Wave  amplitude=1  bias=0  frequency_spec=foundation.enum.frequencySpec.frequencySI  frequency_SI=30 Hz  frequency_angular=1 rad/s  phase=0 rad
      settings: InternalSimscapePortConfiguration="{\"Bottom\":[],\"Left\":[],\"Right\":[{\"id\":\"O\",\"label\":\"\",\"type\":\"output\"}],\"Top\":[]}"
  PS Sine Wave2 : fl_lib/Physical Signals/Sources/PS Sine Wave  amplitude=1  bias=0  frequency_spec=foundation.enum.frequencySpec.frequencySI  frequency_SI=30 Hz  frequency_angular=1 rad/s  phase=2*pi/3+pi/2 rad
      settings: InternalSimscapePortConfiguration="{\"Bottom\":[],\"Left\":[],\"Right\":[{\"id\":\"O\",\"label\":\"\",\"type\":\"output\"}],\"Top\":[]}"
  PS Sine Wave3 : fl_lib/Physical Signals/Sources/PS Sine Wave  amplitude=1  bias=0  frequency_spec=foundation.enum.frequencySpec.frequencySI  frequency_SI=30 Hz  frequency_angular=1 rad/s  phase=2*pi/3 rad
      settings: InternalSimscapePortConfiguration="{\"Bottom\":[],\"Left\":[],\"Right\":[{\"id\":\"O\",\"label\":\"\",\"type\":\"output\"}],\"Top\":[]}"
  PS Sine Wave4 : fl_lib/Physical Signals/Sources/PS Sine Wave  amplitude=1  bias=0  frequency_spec=foundation.enum.frequencySpec.frequencySI  frequency_SI=30 Hz  frequency_angular=1 rad/s  phase=-2*pi/3+pi/2 rad
      settings: InternalSimscapePortConfiguration="{\"Bottom\":[],\"Left\":[],\"Right\":[{\"id\":\"O\",\"label\":\"\",\"type\":\"output\"}],\"Top\":[]}"
  PS Sine Wave5 : fl_lib/Physical Signals/Sources/PS Sine Wave  amplitude=1  bias=0  frequency_spec=foundation.enum.frequencySpec.frequencySI  frequency_SI=30 Hz  frequency_angular=1 rad/s  phase=-2*pi/3 rad
      settings: InternalSimscapePortConfiguration="{\"Bottom\":[],\"Left\":[],\"Right\":[{\"id\":\"O\",\"label\":\"\",\"type\":\"output\"}],\"Top\":[]}"
  aH : PMIOPort  Side=Right
  aL : PMIOPort  Port=2  Side=Right
  bH : PMIOPort  Port=3  Side=Right
  bL : PMIOPort  Port=4  Side=Right
  cH : PMIOPort  Port=5  Side=Right
  cL : PMIOPort  Port=6  Side=Right
  Amp : PMIOPort  Port=7  Side=Left
  connections:
  PS Product5/RConn1 -- cL/RConn1
  PS Product4/RConn1 -- cH/RConn1
  PS Sine Wave5/RConn1 -- PS Math Function5/LConn1
  PS Math Function5/RConn1 -- PS Product5/LConn2
  PS Sine Wave4/RConn1 -- PS Math Function4/LConn1
  PS Math Function4/RConn1 -- PS Product4/LConn2
  PS Product3/RConn1 -- bL/RConn1
  PS Sine Wave3/RConn1 -- PS Math Function3/LConn1
  PS Math Function3/RConn1 -- PS Product3/LConn2
  PS Product2/RConn1 -- bH/RConn1
  PS Sine Wave2/RConn1 -- PS Math Function2/LConn1
  PS Math Function2/RConn1 -- PS Product2/LConn2
  PS Product1/RConn1 -- aL/RConn1
  PS Sine Wave1/RConn1 -- PS Math Function1/LConn1
  PS Math Function1/RConn1 -- PS Product1/LConn2
  PS Sine Wave/RConn1 -- PS Math Function/LConn1
  PS Product4/LConn1 -- PS Product5/LConn1 -- PS Product3/LConn1 -- PS Product2/LConn1 -- PS Product1/LConn1 -- PS Product/LConn1 -- Amp/RConn1
  PS Math Function/RConn1 -- PS Product/LConn2
  aH/RConn1 -- PS Product/RConn1

== system aar_generator/Bus 2/Battery/Subsystem ==
  Internal Resistance : fl_lib/Physical Signals/Sources/PS Constant  constant=0.34 Ohm
  PS Add : fl_lib/Physical Signals/Functions/PS Add
  PS Gain1 : fl_lib/Physical Signals/Functions/PS Gain  gain=0.5
  PS Gain2 : fl_lib/Physical Signals/Functions/PS Gain  gain=battery_cap MW
  PS Gain3 : fl_lib/Physical Signals/Functions/PS Gain  gain=2*350*sqrt(2) kV
  PS Math Function : fl_lib/Physical Signals/Functions/PS Math Function  fcn_choice=foundation.enum.math_function.square  v=1
  PS Math Function1 : fl_lib/Physical Signals/Functions/PS Math Function  fcn_choice=foundation.enum.math_function.reciprocal  v=1
  PS Subtract : fl_lib/Physical Signals/Functions/PS Subtract
  I : PMIOPort  Side=Left
  r : PMIOPort  Port=2  Side=Right
  connections:
  PS Gain3/RConn1 -- PS Subtract/LConn1
  PS Add/LConn1 -- PS Gain2/RConn1
  PS Gain2/LConn1 -- PS Math Function/RConn1
  PS Gain3/LConn1 -- PS Math Function/LConn1 -- PS Math Function1/RConn1
  Internal Resistance/RConn1 -- PS Add/LConn2
  PS Add/RConn1 -- PS Subtract/LConn2
  PS Gain1/RConn1 -- r/RConn1
  PS Gain1/LConn1 -- PS Subtract/RConn1
  I/RConn1 -- PS Math Function1/LConn1

== system aar_generator/Bus 2/Governor and Prime Mover/Governor ==
  pu_velocity : Inport
  1/T_G : Gain  Gain=1/T_G
  1/droop : Gain  Gain=1/(droop_percentage/100)
  Delta load setpoint : Sum  Inputs=+-|
  Delta speed : Sum  Inputs=-+|
  Integrator : Integrator  InitialCondition=pu_torque0
  Load_setpoint : Constant  Value=pu_load_reference_setpoint
  Speed_ref : Constant  Value=pu_speed_reference
  Subtract : Sum  Inputs=|+-
  delta_y : Outport  VectorParamsAs1DForOutWhenUnconnected=off
  wires:
  Integrator/1 -> Subtract/2, delta_y/1
  1/T_G/1 -> Integrator/1
  Subtract/1 -> 1/T_G/1
  Delta load setpoint/1 -> Subtract/1
  1/droop/1 -> Delta load setpoint/2
  pu_velocity/1 -> Delta speed/2
  Load_setpoint/1 -> Delta load setpoint/1
  Delta speed/1 -> 1/droop/1
  Speed_ref/1 -> Delta speed/1

== system aar_generator/Bus 2/Governor and Prime Mover/Non-reheat turbine ==
  delta_y : Inport
  1/T_CH : Gain  Gain=1/T_CH
  Integrator : Integrator  InitialCondition=pu_torque0  UpperSaturationLimit=max_torque
  Max : MinMax  Function=max  Inputs=2
  Min : MinMax  Inputs=2
  Step : Step  Time=contingency_time  Before=max_torque  After=contingency_torque  SampleTime=0
  Sum : Sum  Inputs=|+-
  has_contingency : Constant  Value=max_torque*(1-has_contingency)
  torque : Outport  VectorParamsAs1DForOutWhenUnconnected=off
  wires:
  has_contingency/1 -> Max/1
  Step/1 -> Max/2
  Max/1 -> Min/1
  Integrator/1 -> Min/2
  Min/1 -> torque/1, Sum/2
  1/T_CH/1 -> Integrator/1
  Sum/1 -> 1/T_CH/1
  delta_y/1 -> Sum/1

== system aar_generator/Bus 2/Solar Panel/Current Control ==
  Pset (pu) : Inport
  Qset (pu) : Inport  Port=2
  Phase : Inport  Port=3
  Vabc (pu) : Inport  Port=4
  Constant : Constant  Value=0
  Demux : Demux  Outputs=[2 1]
  Divide : Product  Inputs=*/
  Id : Fcn  Expr=u(1)*u(3)+u(2)*u(4)
  Inverse Park Transform : eeTransforms/Inverse Park Transform  AxisAlignment=Q-axis  PowerInvariant=off
      settings: LibrarySourceBlock=|
      | ee_sl_lib/Mathematical
      | Transforms/Inverse
      | Park Transform
  Iq : Fcn  Expr=u(1)*u(4)-u(2)*u(3)
  Mag^2 : Fcn  Expr=u(1)^2+u(2)^2
  Mux : Mux  Inputs=3
  Mux1 : Mux  Inputs=3
  Park Transform : eeTransforms/Park Transform  AxisAlignment=Q-axis  PowerInvariant=off
      settings: LibrarySourceBlock=|
      | ee_sl_lib/Mathematical
      | Transforms/Park Transform
  Simulink-PS Converter : nesl_utility/Simulink-PS Converter  PhysicalDomain=network_engine_domain  SubClassName=ps_input  LeftPortType=input  RightPortType=output  PseudoPeriodic=off  Frequencies=[]  NoiseDistribution=none  NoiseParameters=[]  Unit=A  AffineConversion=off  FilteringAndDerivatives=filter  SimscapeFilterOrder=1  InputFilterTimeConstant=0.0001  UdotUserProvided=0
  Terminator : Terminator
  Unit Delay1 : UnitDelay  InitialCondition=[0 -sin(2*pi/3) sin(2*pi/3)]  SampleTime=-1  HasFrameUpgradeWarning=on
  pu to SI : Gain  Gain=1/3*0.8*load/350*10^3*sqrt(2)
  Iabc (SI) : PMIOPort  Side=Right
  wires:
  Park Transform/1 -> Demux/1
  Demux/2 -> Terminator/1
  Demux/1 -> Mux/3, Mag^2/1
  Mag^2/1 -> Divide/2
  pu to SI/1 -> Simulink-PS Converter/1
  Constant/1 -> Mux1/3
  Phase/1 -> Inverse Park Transform/2, Park Transform/2
  Vabc (pu)/1 -> Park Transform/1
  Id/1 -> Mux1/1
  Iq/1 -> Mux1/2
  Inverse Park Transform/1 -> Unit Delay1/1
  Unit Delay1/1 -> pu to SI/1
  Mux1/1 -> Divide/1
  Divide/1 -> Inverse Park Transform/1
  Pset (pu)/1 -> Mux/1
  Qset (pu)/1 -> Mux/2
  Mux/1 -> Id/1, Iq/1
  connections:
  Iabc (SI)/RConn1 -- Simulink-PS Converter/RConn1
